simulink model "W02_E_PID"  (R2024b)
settings: Solver=ode4  StartTime=0  StopTime=T_final  FixedStep=h  RelTol=1e-3
values from neighbouring files (symbols this model uses):
  Kd = 4    [W02_0_setup.m]    (also in W02_E_integral.m; W02_I_tuning_by_hand.m = 1)
  Ki = 8    [W02_0_setup.m]
  Kp = 10    [W02_0_setup.m]    (also in W02_D_derivative.m; W02_E_integral.m; W02_I_tuning_by_hand.m = 5*k)
  Nf = 20    [W02_0_setup.m]    (also in W02_G_lowpass_filter.m = Nf(i))
  pid_b = 2    [W02_0_setup.m]
  pid_k = 2    [W02_0_setup.m]
  pid_m = 1    [W02_0_setup.m]
  t_step = 1    [W02_0_setup.m]
  y_step = 1    [W02_0_setup.m]
settings Model: Creator=admin  LastModifiedBy=admin
settings DataIOCC: ReturnWorkspaceOutputs=off

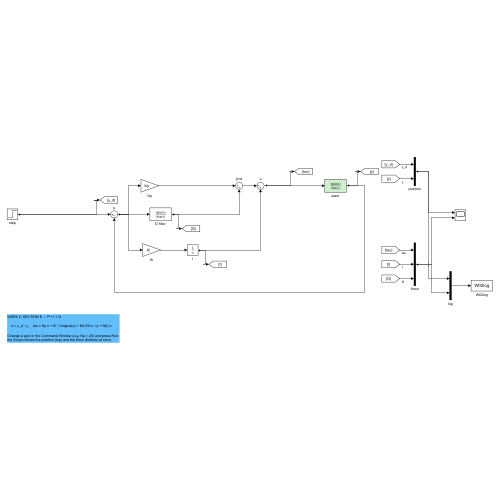
[thumbnail: Simulink's stored preview of the top-level diagram]
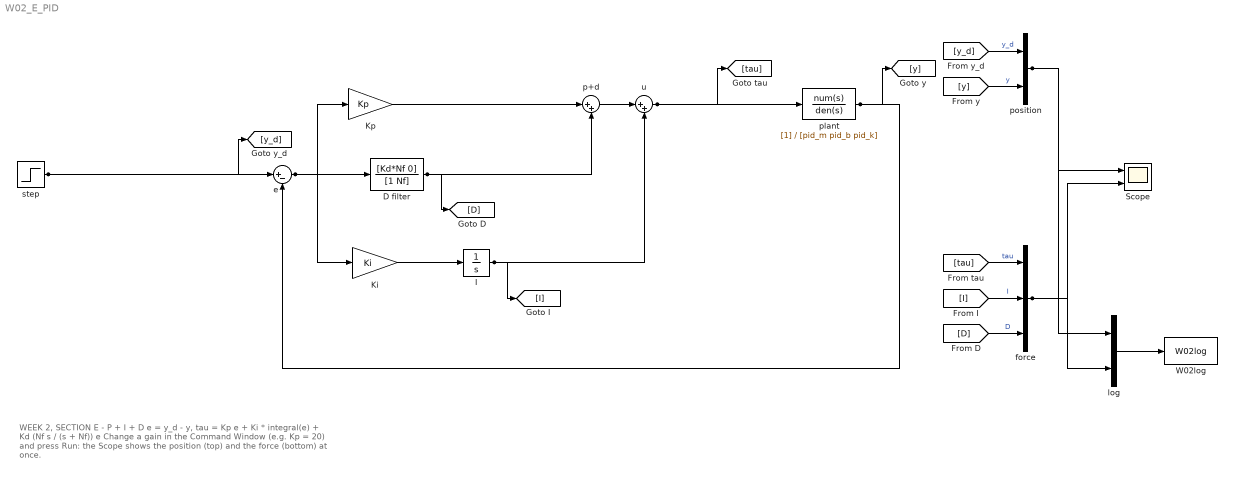
== system W02_E_PID ==
  note: WEEK 2, SECTION E  -  P + I + D
      |
      |     e = y_d - y,    tau = Kp e + Ki * integral(e) + Kd (Nf s / (s + Nf)) e
      |
      | Change a gain in the Command Window (e.g. Kp = 20) and press Run:
      | the Scope shows the position (top) and the force (bottom) at once.
  D filter : TransferFcn  Numerator=[Kd*Nf 0]  Denominator=[1 Nf]
  I : Integrator
  Ki : Gain  Gain=Ki
  Kp : Gain  Gain=Kp
  Scope : Scope  NumInputPorts=2
  W02log : ToWorkspace  VariableName=W02log  SaveFormat=Structure With Time  SampleTime=-1
  e : Sum  Inputs=|+-
  force : Mux  Inputs=3
  log : Mux  Inputs=2
  p+d : Sum  Inputs=|++
  plant : TransferFcn  Denominator=[pid_m pid_b pid_k]
  position : Mux  Inputs=2
  step : Step  Time=t_step  After=y_step  SampleTime=0
  u : Sum  Inputs=|++
  wires:
  step/1 -> e/1, [y_d]
  e/1 -> Kp/1, D filter/1, Ki/1
  Kp/1 -> p+d/1
  D filter/1 -> p+d/2, [D]
  Ki/1 -> I/1
  p+d/1 -> u/1
  I/1 -> u/2, [I]
  u/1 -> plant/1, [tau]
  plant/1 -> [y], e/2
  [y_d] -> position/1  "y_d"
  [y] -> position/2  "y"
  [tau] -> force/1  "tau"
  [I] -> force/2  "I"
  [D] -> force/3  "D"
  position/1 -> Scope/1, log/1
  force/1 -> Scope/2, log/2
  log/1 -> W02log/1
